simulink model "sampleModel1499"  (R2023a)
settings: Solver=VariableStepAuto  StartTime=0.0  StopTime=10.0  RelTol=1e-3
libraries: hdlsllib x4, simulink x1
settings Model: Creator=user1  LastModifiedBy=user1

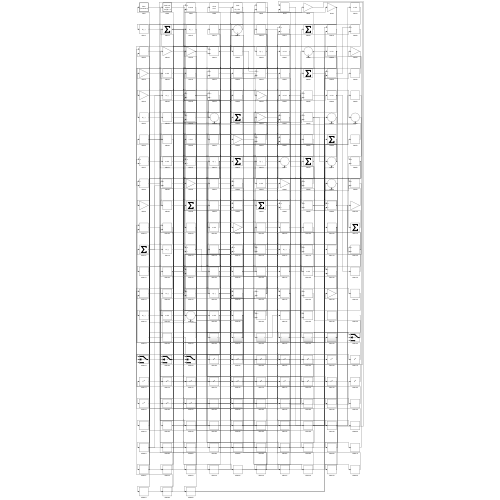
[thumbnail: Simulink's stored preview of the top-level diagram]
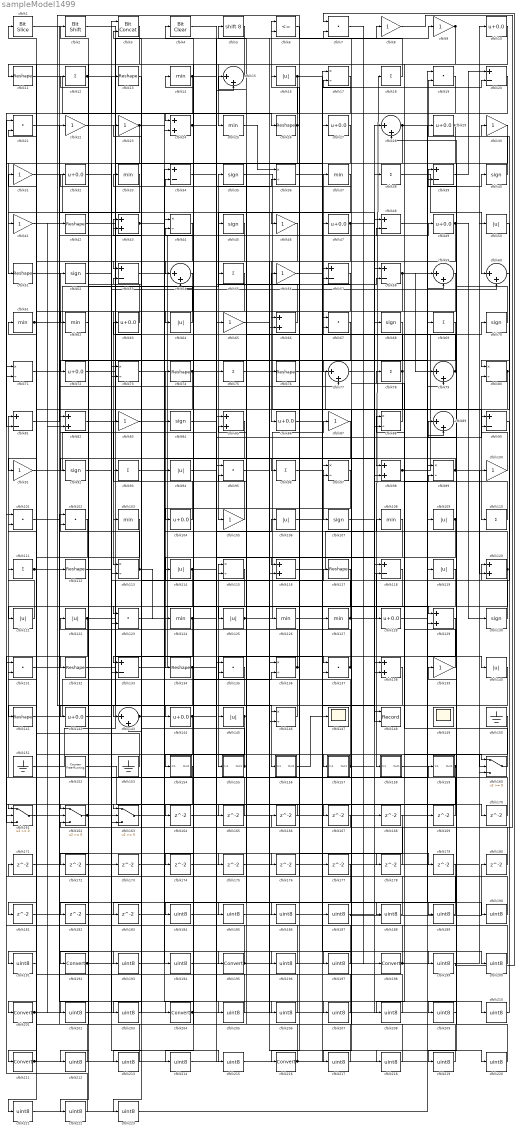
== system sampleModel1499 ==
  cfblk1 : hdlsllib/Logic and Bit Operations/Bit Slice  lidx=7  ridx=0
  cfblk{10,27,29,32,47,49,63,72,86,104,128,142,144} (13 alike) : Bias  Bias=0.0  SaturateOnIntegerOverflow=off
  cfblk{8..9,22..23,30..31,41,46,56,65,83,87,91,100,105,139} (16 alike) : Gain
  cfblk{7,19,21,67,95,101..102,123,131,135,137} (11 alike) : DotProduct  OutDataTypeStr=Inherit: Inherit via internal rule
  cfblk{14,25,33,37,61..62,103,108,124,126..127} (11 alike) : MinMax
  cfblk{16,50,64,94,106,109,114,119,121..122,125,140,145} (13 alike) : Abs  SaturateOnIntegerOverflow=off
  cfblk{35,40,45,52,68,70,84,92,107,130} (10 alike) : Signum
  cfblk{11,13,26,42,51,74,76,112,117,132,134,141} (12 alike) : Reshape
  cfblk{12,18,38,55,69,75,78,93,96,110..111} (11 alike) : Sum  Inputs=+
  cfblk{17,36,44,71,73,80,88,97,99,113,115,136,146} (13 alike) : Product  Inputs=*/  RndMeth=Zero  SaturateOnIntegerOverflow=on
  cfblk{24,43,66,82,85,98,116,120,129,138} (10 alike) : Sum
  cfblk{20,34,39,48,53,57..58,81,90,118,133} (11 alike) : Sum  Inputs=+-
  cfblk{15,28,54,59..60,77,79,89,143} (9 alike) : Sum  Inputs=|++
  cfblk147 : Scope
  cfblk148 : Record  FileSettingsInternal="{\"entries\":[{\"content\":{\"excelSettings\":{\"content\":{},\"type\":\"Streamout.ExcelSettings\"}},\"type\":\"Streamout.FileSettingStorage\",\"uuid\":\"\"}],\"packageUris\":[\"http:\\/\\/schema.mathworks.com\\/mf0\\/streamout_blocks\\/R2020a\"],\"version\":\"1.0\"}"  Layout=[1 1]  SignalsInternal="{\"entries\":[{\"content\":{\"signals\":[{\"content\":{\"blockPath\":[],\"dimensions\":[1],\"domain\":\"\",\"lineColor\":\"#a2142f\",\"plots\":[1],\"port\":1,\"signalID\":1259,\"signalName\":\"XY Graph:1\"},\"type\":\"RecordBlkView.Signal\",\"uuid\":\"\"},{\"content\":{\"blockPath\":[],\"dimensions\":[1],\"domain\":\"\",\"lineColor\":\"#139fff\",\"plots\":[1],\"port\":2,\"signalID\":1262,\"signalName\":\"XY Graph:2\"},\"type\":\"RecordBlkView.Signal\",\"uuid\":\"\"}]},\"type\":\"RecordBlkView.InputSignals\",\"uuid\":\"\"}],\"packageUris\":[\"http:\\/\\/schema.mathworks.com\\/mf0\\/streamout_blocks\\/R2020a\"],\"version\":\"1.0\"}"  VisualizationBindings="{\"xyplotplugin\":{\"info\":[{\"series\":[{\"bindingParametersList\":[{\"parameter\":\"X-Axis\",\"signalID\":1259,\"signalName\":\"XY Graph:1\"},{\"parameter\":\"Y-Axis\",\"signalID\":1262,\"signalName\":\"XY Graph:2\"}],\"seriesID\":9767}],\"subplotID\":1}]}}"  CompatibilityTag=XY  st=-1
  cfblk149 : Scope
      settings: Floating=on
  cfblk150 : Ground
  cfblk151 : Ground
  cfblk152 : hdlsllib/Sources/Counter Free-Running  NumBits=16  tsamp=-1
  cfblk153 : Ground
  cfblk154 : Subsystem
      settings: LibrarySourceBlock=|
      | hdlsllib/Ports &
      | Subsystems/Subsystem
  cfblk155 : Subsystem
      settings: LibrarySourceBlock=|
      | hdlsllib/Ports &
      | Subsystems/Subsystem
  cfblk156 : Subsystem
      settings: LibrarySourceBlock=|
      | hdlsllib/Ports &
      | Subsystems/Subsystem
  cfblk157 : Subsystem
      settings: LibrarySourceBlock=|
      | hdlsllib/Ports &
      | Subsystems/Subsystem
  cfblk158 : Subsystem
      settings: LibrarySourceBlock=|
      | hdlsllib/Ports &
      | Subsystems/Subsystem
  cfblk159 : Subsystem
      settings: LibrarySourceBlock=|
      | hdlsllib/Ports &
      | Subsystems/Subsystem
  cfblk{160..163} (4 alike) : Switch  SaturateOnIntegerOverflow=off  InputSameDT=off
  cfblk{164..183} (20 alike) : Delay  SampleTime=1
  cfblk{184..191,193..194,196..197,199..200,202..203,205..210,212..215,217..223} (33 alike) : DataTypeConversion  OutDataTypeStr=uint8  SaturateOnIntegerOverflow=off  RndMeth=Floor
  cfblk{192,195,198,201,204,211,216} (7 alike) : DataTypeConversion  SaturateOnIntegerOverflow=off  RndMeth=Floor
  cfblk2 : hdlsllib/Logic and Bit Operations/Bit Shift  mode=Shift Left Logical  N=0
  cfblk3 : hdlsllib/Logic and Bit Operations/Bit Concat  numInputs=2
  cfblk4 : simulink/Logic and Bit Operations/Bit Clear  iBit=0
      settings: LibrarySourceBlock=|
      | hdlsllib/Logic and Bit
      | Operations/Bit Clear
  cfblk5 : ArithShift  BitShiftNumber=8
  cfblk6 : RelationalOperator  Operator=<=  OutDataTypeStr=boolean  InputSameDT=off
  wires:
  cfblk82/1 -> cfblk6/1
  cfblk133/1 -> cfblk49/1
  cfblk157/1(Out1) -> cfblk115/1, cfblk99/2
  cfblk113/1 -> cfblk52/1, cfblk124/1
  cfblk156/1(Out1) -> cfblk147/1
  cfblk108/1 -> cfblk158/1(In1)
  cfblk151/1 -> cfblk74/1
  cfblk125/1 -> cfblk87/1, cfblk8/1
  cfblk57/1 -> cfblk154/1(In1)
  cfblk120/1 -> cfblk84/1, cfblk14/1, cfblk208/1
  cfblk127/1 -> cfblk18/1, cfblk63/1
  cfblk18/1 -> cfblk143/1
  cfblk25/1 -> cfblk36/1
  cfblk7/1 -> cfblk198/1
  cfblk46/1 -> cfblk86/1
  cfblk38/1 -> cfblk60/1
  cfblk150/1 -> cfblk81/1
  cfblk50/1 -> cfblk80/1
  cfblk119/1 -> cfblk121/1
  cfblk9/1 -> cfblk25/1, cfblk128/1
  cfblk86/1 -> cfblk27/1
  cfblk12/1 -> cfblk155/1(In1), cfblk24/1, cfblk24/2
  cfblk2/1 -> cfblk156/1(In1)
  cfblk76/1 -> cfblk98/1
  cfblk90/1 -> cfblk120/1
  cfblk37/1 -> cfblk105/1
  cfblk39/1 -> cfblk20/1
  cfblk130/1 -> cfblk94/1
  cfblk54/1 -> cfblk113/1
  cfblk19/1 -> cfblk81/2
  cfblk66/1 -> cfblk35/1
  cfblk16/1 -> cfblk146/1, cfblk142/1, cfblk160/2
  cfblk73/1 -> cfblk98/2
  cfblk132/1 -> cfblk115/2
  cfblk160/1 -> cfblk78/1
  cfblk74/1 -> cfblk103/1, cfblk34/2, cfblk57/1, cfblk123/2, cfblk191/1
  cfblk88/1 -> cfblk33/1
  cfblk35/1 -> cfblk110/1
  cfblk129/1 -> cfblk145/1
  cfblk81/1 -> cfblk22/1
  cfblk3/1 -> cfblk201/1
  cfblk102/1 -> cfblk211/1
  cfblk22/1 -> cfblk127/1
  cfblk15/1 -> cfblk11/1
  cfblk59/1 -> cfblk132/1
  cfblk42/1 -> cfblk77/1
  cfblk109/1 -> cfblk134/1, cfblk116/1
  cfblk13/1 -> cfblk163/1
  cfblk105/1 -> cfblk23/1
  cfblk162/1 -> cfblk82/1, cfblk136/2, cfblk159/1(In1)
  cfblk163/1 -> cfblk119/1
  cfblk118/1 -> cfblk123/1
  cfblk51/1 -> cfblk45/1
  cfblk80/1 -> cfblk125/1, cfblk167/1
  cfblk33/1 -> cfblk51/1
  cfblk96/1 -> cfblk107/1
  cfblk98/1 -> cfblk50/1, cfblk40/1
  cfblk144/1 -> cfblk90/2, cfblk183/1
  cfblk17/1 -> cfblk216/1
  cfblk31/1 -> cfblk148/1
  cfblk107/1 -> cfblk68/1
  cfblk79/1 -> cfblk37/1, cfblk5/1
  cfblk20/1 -> cfblk64/1
  cfblk116/1 -> cfblk58/1
  cfblk128/1 -> cfblk19/1
  cfblk53/1 -> cfblk47/1
  cfblk14/1 -> cfblk172/1, cfblk210/1
  cfblk40/1 -> cfblk19/2
  cfblk32/1 -> cfblk144/1
  cfblk11/1 -> cfblk65/1
  cfblk23/1 -> cfblk41/1, cfblk176/1
  cfblk47/1 -> cfblk118/1, cfblk116/2
  cfblk10/1 -> cfblk72/1
  cfblk72/1 -> cfblk70/1
  cfblk5/1 -> cfblk54/1
  cfblk58/1 -> cfblk140/1, cfblk104/1, cfblk79/1
  cfblk67/1 -> cfblk96/1
  cfblk64/1 -> cfblk2/1
  cfblk137/1 -> cfblk53/2, cfblk197/1
  cfblk99/1 -> cfblk120/2, cfblk92/1
  cfblk142/1 -> cfblk117/1
  cfblk24/1 -> cfblk26/1, cfblk54/2
  cfblk110/1 -> cfblk88/1
  cfblk29/1 -> cfblk113/2, cfblk53/1, cfblk185/1
  cfblk124/1 -> cfblk133/1, cfblk36/2
  cfblk41/1 -> cfblk77/2
  cfblk65/1 -> cfblk126/1
  cfblk55/1 -> cfblk141/1
  cfblk139/1 -> cfblk108/1
  cfblk100/1 -> cfblk80/2
  cfblk145/1 -> cfblk163/2, cfblk181/1
  cfblk28/1 -> cfblk73/2, cfblk190/1
  cfblk143/1 -> cfblk160/1, cfblk206/1
  cfblk1/1 -> cfblk46/1
  cfblk138/1 -> cfblk146/2
  cfblk158/1(Out1) -> cfblk59/2
  cfblk27/1 -> cfblk71/2
  cfblk49/1 -> cfblk91/1, cfblk130/1
  cfblk122/1 -> cfblk137/1, cfblk161/3, cfblk60/2
  cfblk61/1 -> cfblk55/1, cfblk109/1
  cfblk85/1 -> cfblk204/1
  cfblk77/1 -> cfblk88/2
  cfblk136/1 -> cfblk15/1, cfblk16/1, cfblk32/1
  cfblk134/1 -> cfblk9/1, cfblk163/3, cfblk106/1
  cfblk91/1 -> cfblk75/1
  cfblk114/1 -> cfblk67/1, cfblk157/1(In1), cfblk58/2, cfblk161/1
  cfblk104/1 -> cfblk83/1
  cfblk146/1 -> cfblk4/1
  cfblk135/1 -> cfblk162/2
  cfblk21/1 -> cfblk195/1
  cfblk159/1(Out1) -> cfblk39/1, cfblk161/2
  cfblk155/1(Out1) -> cfblk43/1, cfblk43/2
  cfblk75/1 -> cfblk99/1
  cfblk112/1 -> cfblk133/2
  cfblk60/1 -> cfblk90/1
  cfblk70/1 -> cfblk28/2
  cfblk44/1 -> cfblk192/1
  cfblk126/1 -> cfblk48/2
  cfblk63/1 -> cfblk12/1
  cfblk48/1 -> cfblk29/1
  cfblk43/1 -> cfblk34/1, cfblk129/1
  cfblk106/1 -> cfblk148/2
  cfblk153/1 -> cfblk61/1
  cfblk111/1 -> cfblk112/1, cfblk82/2
  cfblk121/1 -> cfblk111/1
  cfblk36/1 -> cfblk20/2
  cfblk78/1 -> cfblk57/2, cfblk221/1
  cfblk84/1 -> cfblk118/2
  cfblk26/1 -> cfblk6/2, cfblk62/1
  cfblk6/1 -> cfblk66/1
  cfblk141/1 -> cfblk13/1
  cfblk45/1 -> cfblk164/1
  cfblk164/1 -> cfblk28/1
  cfblk87/1 -> cfblk165/1
  cfblk165/1 -> cfblk1/1
  cfblk8/1 -> cfblk166/1
  cfblk166/1 -> cfblk162/1
  cfblk167/1 -> cfblk162/3
  cfblk169/1 -> cfblk67/2
  cfblk123/1 -> cfblk170/1
  cfblk170/1 -> cfblk71/1
  cfblk171/1 -> cfblk137/2
  cfblk172/1 -> cfblk160/3
  cfblk92/1 -> cfblk173/1
  cfblk173/1 -> cfblk143/2
  cfblk140/1 -> cfblk174/1
  cfblk83/1 -> cfblk175/1
  cfblk94/1 -> cfblk178/1
  cfblk178/1 -> cfblk48/1
  cfblk161/1 -> cfblk179/1
  cfblk180/1 -> cfblk95/2
  cfblk181/1 -> cfblk136/1
  cfblk62/1 -> cfblk182/1
  cfblk182/1 -> cfblk138/2
  cfblk183/1 -> cfblk135/1
  cfblk97/1 -> cfblk184/1
  cfblk184/1 -> cfblk138/1
  cfblk185/1 -> cfblk97/1
  cfblk168/1 -> cfblk186/1
  cfblk186/1 -> cfblk97/2
  cfblk56/1 -> cfblk187/1
  cfblk187/1 -> cfblk180/1
  cfblk34/1 -> cfblk188/1
  cfblk188/1 -> cfblk56/1
  cfblk101/1 -> cfblk189/1
  cfblk189/1 -> cfblk95/1
  cfblk190/1 -> cfblk101/1
  cfblk191/1 -> cfblk101/2
  cfblk192/1 -> cfblk38/1, cfblk10/1
  cfblk71/1 -> cfblk193/1
  cfblk193/1 -> cfblk44/1
  cfblk152/1 -> cfblk194/1
  cfblk194/1 -> cfblk44/2
  cfblk195/1 -> cfblk76/1, cfblk39/2, cfblk73/1
  cfblk174/1 -> cfblk196/1
  cfblk196/1 -> cfblk21/1
  cfblk197/1 -> cfblk21/2
  cfblk198/1 -> cfblk129/2, cfblk100/1, cfblk79/2, cfblk122/1
  cfblk4/1 -> cfblk199/1
  cfblk199/1 -> cfblk7/1
  cfblk176/1 -> cfblk200/1
  cfblk200/1 -> cfblk7/2
  cfblk201/1 -> cfblk169/1, cfblk42/1
  cfblk103/1 -> cfblk202/1
  cfblk202/1 -> cfblk3/1
  cfblk115/1 -> cfblk203/1
  cfblk203/1 -> cfblk3/2
  cfblk204/1 -> cfblk168/1, cfblk66/2
  cfblk131/1 -> cfblk205/1
  cfblk205/1 -> cfblk85/1
  cfblk206/1 -> cfblk85/2
  cfblk93/1 -> cfblk207/1
  cfblk207/1 -> cfblk171/1
  cfblk208/1 -> cfblk93/1
  cfblk30/1 -> cfblk209/1
  cfblk209/1 -> cfblk139/1
  cfblk210/1 -> cfblk30/1
  cfblk211/1 -> cfblk131/2, cfblk59/1
  cfblk117/1 -> cfblk212/1
  cfblk212/1 -> cfblk102/1
  cfblk68/1 -> cfblk213/1
  cfblk213/1 -> cfblk102/2
  cfblk177/1 -> cfblk214/1
  cfblk214/1 -> cfblk15/2
  cfblk52/1 -> cfblk215/1
  cfblk215/1 -> cfblk177/1
  cfblk216/1 -> cfblk31/1, cfblk135/2
  cfblk179/1 -> cfblk217/1
  cfblk217/1 -> cfblk17/1
  cfblk95/1 -> cfblk218/1
  cfblk218/1 -> cfblk17/2
  cfblk89/1 -> cfblk219/1
  cfblk219/1 -> cfblk114/1
  cfblk175/1 -> cfblk220/1
  cfblk220/1 -> cfblk89/1
  cfblk221/1 -> cfblk89/2
  cfblk69/1 -> cfblk222/1
  cfblk222/1 -> cfblk131/1
  cfblk154/1(Out1) -> cfblk223/1
  cfblk223/1 -> cfblk69/1

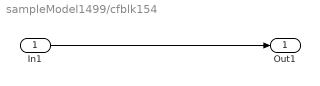
== system sampleModel1499/cfblk154 ==
  In1 : Inport
  Out1 : Outport
  wires:
  In1/1 -> Out1/1

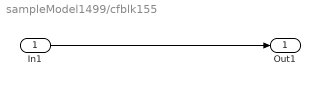
== system sampleModel1499/cfblk155 ==
  In1 : Inport
  Out1 : Outport
  wires:
  In1/1 -> Out1/1

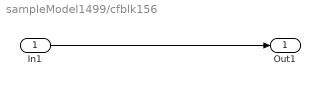
== system sampleModel1499/cfblk156 ==
  In1 : Inport
  Out1 : Outport
  wires:
  In1/1 -> Out1/1

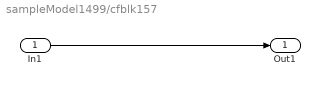
== system sampleModel1499/cfblk157 ==
  In1 : Inport
  Out1 : Outport
  wires:
  In1/1 -> Out1/1

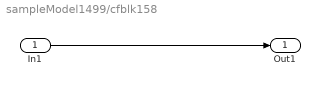
== system sampleModel1499/cfblk158 ==
  In1 : Inport
  Out1 : Outport
  wires:
  In1/1 -> Out1/1

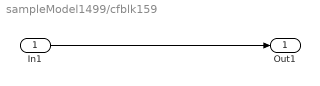
== system sampleModel1499/cfblk159 ==
  In1 : Inport
  Out1 : Outport
  wires:
  In1/1 -> Out1/1
